simulink model "exnb4137986_Q6"  (R2023b)
settings: Solver=FixedStepAuto  StartTime=0.0  StopTime=200  FixedStep=0.01  RelTol=1e-3
values from neighbouring files (symbols this model uses):
  C = [1, 0]    [exnb4137986_Q6_par.m]
  equ_1 = [u_star_1, x_star_1]    [exnb4137986_Q5_par.m]    (also in exnb4137986_Q6_par.m)
  equ_2 = [u_star_2, x_star_2]    [exnb4137986_Q5_par.m]    (also in exnb4137986_Q6_par.m)
  K = place(A, B, lambda_cl)    [exnb4137986_Q5_par.m]    (also in exnb4137986_Q6_par.m)
  Ki = lqi(sys_CT,Q,R)    [exnb4137986_Q6_par.m]
  values = [0.005, 10]    [exnb4137986_Q3_par.m]    (also in exnb4137986_Q5_par.m; exnb4137986_Q6_par.m)
settings Model: Creator=therkelsen  LastModifiedBy=therkelsen

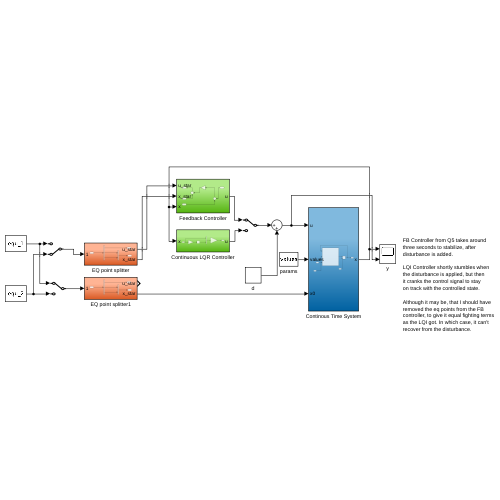
[thumbnail: Simulink's stored preview of the top-level diagram]
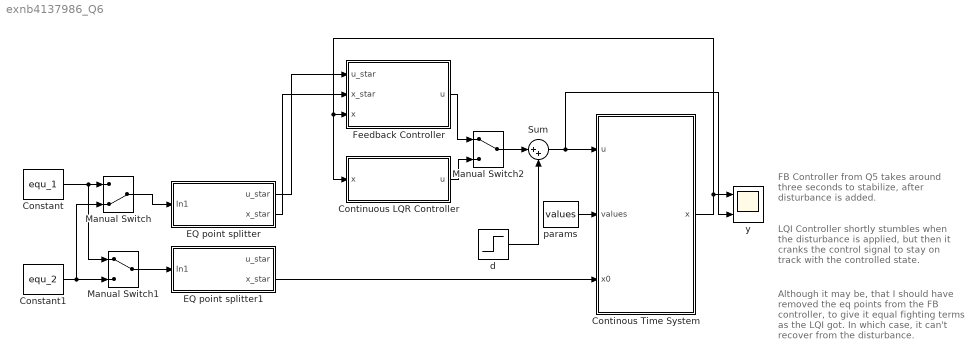
== system exnb4137986_Q6 ==
  note: Although it may be, that I should have
      | removed the eq points from the FB
      | controller, to give it equal fighting terms
      | as the LQI got. In which case, it can't
      | recover from the disturbance.
  note: LQI Controller shortly stumbles when
      | the disturbance is applied, but then
      | it cranks the control signal to stay
      | on track with the controlled state.
  note: FB Controller from Q5 takes around
      | three seconds to stabilize, after
      | disturbance is added.
  Constant : Constant  Value=equ_1
  Constant1 : Constant  Value=equ_2
  Continous Time System : Subsystem
  Continuous LQR Controller : Subsystem
  EQ point splitter : Subsystem
  EQ point splitter1 : Subsystem
  Feedback Controller : Subsystem
  Manual Switch : ManualSwitch  CurrentSetting=0
  Manual Switch1 : ManualSwitch
  Manual Switch2 : ManualSwitch
  Sum : Sum  Inputs=|++
  d : Step  Time=3  After=-10  SampleTime=0
  params : Constant  Value=values
  y : Scope  NumInputPorts=2
  wires:
  Continous Time System/1(x) -> Continuous LQR Controller/1(x), Feedback Controller/3(x), y/1
  Sum/1 -> y/2, Continous Time System/1(u)
  params/1 -> Continous Time System/2(values)
  Manual Switch/1 -> EQ point splitter/1(In1)
  Constant1/1 -> Manual Switch/2, Manual Switch1/2
  Constant/1 -> Manual Switch1/1, Manual Switch/1
  Manual Switch1/1 -> EQ point splitter1/1(In1)
  EQ point splitter1/2(x_star) -> Continous Time System/3(x0)
  d/1 -> Sum/2
  Manual Switch2/1 -> Sum/1
  Feedback Controller/1(u) -> Manual Switch2/1
  Continuous LQR Controller/1(u) -> Manual Switch2/2
  EQ point splitter/1(u_star) -> Feedback Controller/1(u_star)
  EQ point splitter/2(x_star) -> Feedback Controller/2(x_star)

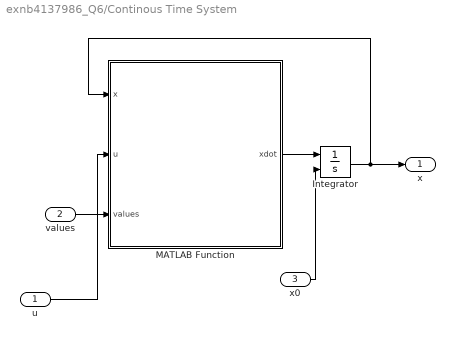
== system exnb4137986_Q6/Continous Time System ==
  u : Inport
  values : Inport  Port=2
  x0 : Inport  Port=3
  Integrator : Integrator  InitialConditionSource=external
  MATLAB Function : MATLAB Function  TreatAsAtomicUnit=on
  x : Outport
  wires:
  MATLAB Function/1(xdot) -> Integrator/1
  values/1 -> MATLAB Function/3(values)
  u/1 -> MATLAB Function/2(u)
  x0/1 -> Integrator/2
  Integrator/1 -> x/1, MATLAB Function/1(x)

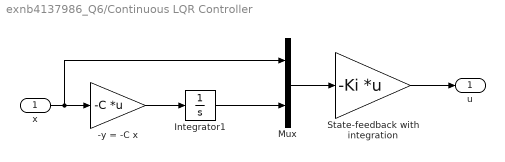
== system exnb4137986_Q6/Continuous LQR Controller ==
  x : Inport
  -y = -C x : Gain  Gain=-C  Multiplication=Matrix(K*u) (u vector)
  Integrator1 : Integrator
  Mux : Mux  Inputs=2
  State-feedback with integration : Gain  Gain=-Ki  Multiplication=Matrix(K*u) (u vector)
  u : Outport
  wires:
  x/1 -> Mux/1, -y = -C x/1
  -y = -C x/1 -> Integrator1/1
  Integrator1/1 -> Mux/2
  Mux/1 -> State-feedback with integration/1
  State-feedback with integration/1 -> u/1

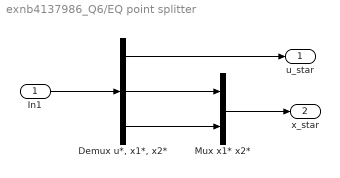
== system exnb4137986_Q6/EQ point splitter ==
  In1 : Inport
  "Demux u*, x1*, x2*" : Demux  Outputs=3
  Mux x1* x2* : Mux  Inputs=2
  u_star : Outport
  x_star : Outport  Port=2
  wires:
  "Demux u*, x1*, x2*"/3 -> Mux x1* x2*/2
  Mux x1* x2*/1 -> x_star/1
  "Demux u*, x1*, x2*"/2 -> Mux x1* x2*/1
  "Demux u*, x1*, x2*"/1 -> u_star/1
  In1/1 -> "Demux u*, x1*, x2*"/1

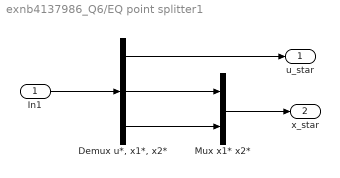
== system exnb4137986_Q6/EQ point splitter1 ==
  In1 : Inport
  "Demux u*, x1*, x2*" : Demux  Outputs=3
  Mux x1* x2* : Mux  Inputs=2
  u_star : Outport
  x_star : Outport  Port=2
  wires:
  "Demux u*, x1*, x2*"/3 -> Mux x1* x2*/2
  Mux x1* x2*/1 -> x_star/1
  "Demux u*, x1*, x2*"/2 -> Mux x1* x2*/1
  "Demux u*, x1*, x2*"/1 -> u_star/1
  In1/1 -> "Demux u*, x1*, x2*"/1

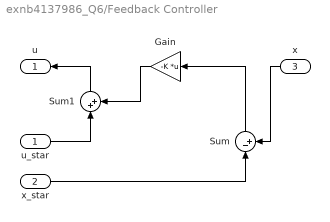
== system exnb4137986_Q6/Feedback Controller ==
  u_star : Inport
  x_star : Inport  Port=2
  x : Inport  Port=3
  Gain : Gain  Gain=-K  Multiplication=Matrix(K*u)
  Sum : Sum  Inputs=|-+
  Sum1 : Sum  Inputs=|++
  u : Outport
  wires:
  x/1 -> Sum/2
  Gain/1 -> Sum1/2
  Sum/1 -> Gain/1
  x_star/1 -> Sum/1
  u_star/1 -> Sum1/1
  Sum1/1 -> u/1

== matlab function exnb4137986_Q6/Continous Time System/MATLAB Function ==
  data: x input; u input; xdot output; values input
function xdot = fcn(x, u, values)

d = values(1);
lambda = values(2);

xdot = [-d*x(1)*abs(x(1)) + x(2);
         -lambda*x(2) + u];
